simulink model "sim_0_spring_mass_model"  (R2021a)
settings: Solver=ode45  StartTime=0.0  StopTime=10.0  RelTol=1e-7
settings Model: Creator=bhorton  LastModifiedBy=Petronas-Tareq
settings SolverCC: AlgebraicLoopSolver=TrustRegion
settings DataIOCC: ReturnWorkspaceOutputs=off
settings DebuggingCC: SFMachineParentedDataDiag=warning  ArithmeticOperatorsInVariantConditions=warning
settings SFSimCC: SimUseLocalCustomCode=off  CustomCodeUndefinedFunction=UseInterfaceOnly
settings RTWCC: RTWUseLocalCustomCode=off
settings CodeAppCC: StateflowObjectComments=on

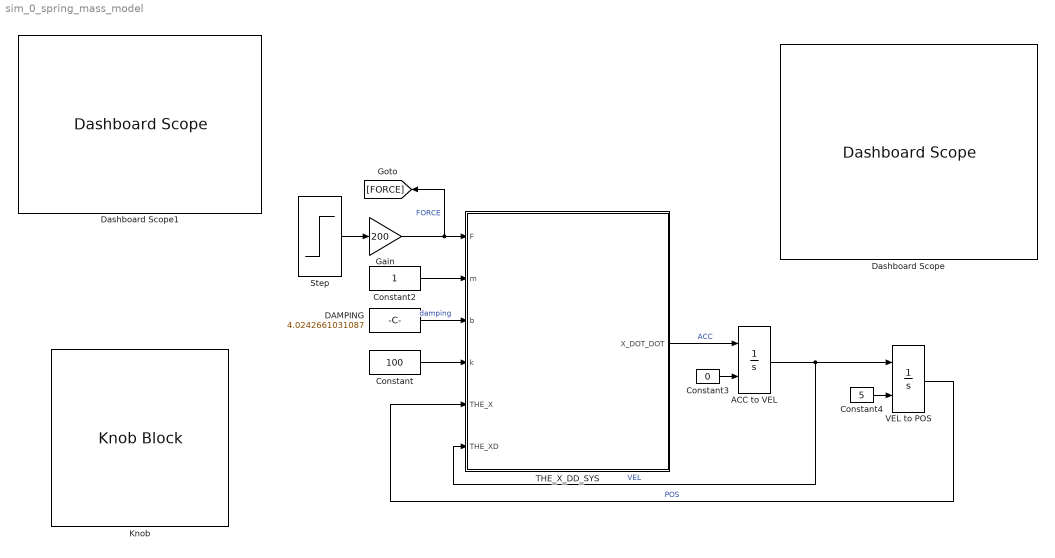
== system sim_0_spring_mass_model ==
  ACC to VEL : Integrator  InitialConditionSource=external
  Constant : Constant  Value=100
  Constant2 : Constant
  Constant3 : Constant  Value=0
  Constant4 : Constant  Value=5
  DAMPING : Constant  Value=4.0242661031087
  Dashboard Scope : DashboardScope
  Dashboard Scope1 : DashboardScope
  Gain : Gain  Gain=200
  Knob : KnobBlock  ScaleMin=1  ScaleMax=15
  Step : Step  Time=5  SampleTime=0
  THE_X_DD_SYS : MATLAB Function  TreatAsAtomicUnit=on
  VEL to POS : Integrator  InitialConditionSource=external
  wires:
  Step/1 -> Gain/1
  Gain/1 -> THE_X_DD_SYS/1(F), [FORCE]  "FORCE"
  THE_X_DD_SYS/1(X_DOT_DOT) -> ACC to VEL/1  "ACC"
  ACC to VEL/1 -> THE_X_DD_SYS/6(THE_XD), VEL to POS/1  "VEL"
  VEL to POS/1 -> THE_X_DD_SYS/5(THE_X)  "POS"
  Constant2/1 -> THE_X_DD_SYS/2(m)
  DAMPING/1 -> THE_X_DD_SYS/3(b)  "damping"
  Constant/1 -> THE_X_DD_SYS/4(k)
  Constant3/1 -> ACC to VEL/2
  Constant4/1 -> VEL to POS/2

== matlab function sim_0_spring_mass_model/THE_X_DD_SYS ==
  data: F input; X_DOT_DOT output; m input; b input; k input; THE_X input; THE_XD input
function X_DOT_DOT = THE_X_DD_SYS(F,m,b,k,THE_X,THE_XD)
%#codegen

%    This function was generated by the Symbolic Math Toolbox version 7.2.
%    27-Mar-2017 09:20:04

X_DOT_DOT = -(-F+THE_XD.*b+THE_X.*k)./m;
